simulink model "Sphase"  (R2017a)
settings: Solver=FixedStepDiscrete  StartTime=0.0  StopTime=0.125 - 5e-5  MaxStep=1e-4  RelTol=1e-3
libraries: powerlib x12, auto_lib x2
settings Model: Creator=ioanna  LastModifiedBy=ioanna

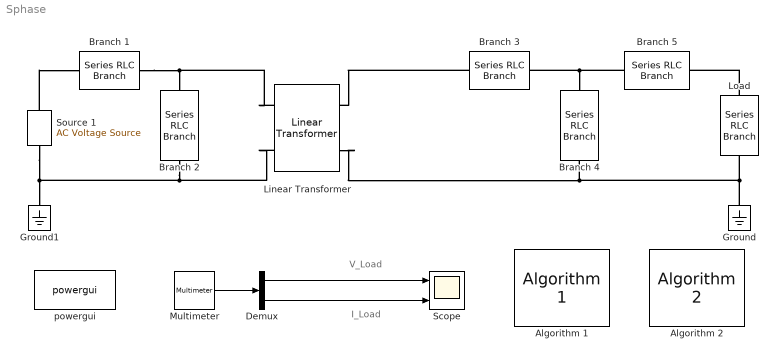
== system Sphase ==
  note: I_Load
  note: V_Load
  Algorithm 1 : auto_lib/Algorithm 1  SystemSampleTime=-1
      settings: SourceProductName=Auto_Design_Framework
  Algorithm 2 : auto_lib/Algorithm 2  SystemSampleTime=-1
      settings: SourceProductName=Auto_Design_Framework
  Branch 1 : powerlib/Elements/Series RLC Branch  LConnTagsString=__new0  RConnTagsString=__new0  BranchType=R  Resistance=5  Inductance=0.02  SetiL0=off  InitialCurrent=0  Capacitance=1e-6  Setx0=off  InitialVoltage=0  Measurements=None
  Branch 2 : powerlib/Elements/Series RLC Branch  LConnTagsString=__new0  RConnTagsString=__new0  BranchType=RC  Resistance=5  Inductance=0.02  SetiL0=off  InitialCurrent=0  Capacitance=1e-4  Setx0=off  InitialVoltage=0  Measurements=None
  Branch 3 : powerlib/Elements/Series RLC Branch  LConnTagsString=__new0  RConnTagsString=__new0  BranchType=R  Resistance=5  Inductance=0.02  SetiL0=off  InitialCurrent=0  Capacitance=1e-6  Setx0=off  InitialVoltage=0  Measurements=None
  Branch 4 : powerlib/Elements/Series RLC Branch  LConnTagsString=__new0  RConnTagsString=__new0  BranchType=RC  Resistance=5  Inductance=0.02  SetiL0=off  InitialCurrent=0  Capacitance=1e-4  Setx0=off  InitialVoltage=0  Measurements=None
  Branch 5 : powerlib/Elements/Series RLC Branch  LConnTagsString=__new0  RConnTagsString=__new0  BranchType=RL  Resistance=5  Inductance=0.02  SetiL0=off  InitialCurrent=0  Capacitance=1e-6  Setx0=off  InitialVoltage=0  Measurements=None
  Demux : Demux  Outputs=2
  Ground : powerlib/Elements/Ground  LConnTagsString=a
  Ground1 : powerlib/Elements/Ground  LConnTagsString=a
  Linear Transformer : powerlib/Elements/Linear Transformer  UNITS=SI  NominalPower=[5e3 50]  winding1=[220 0.5 0.001]  winding2=[440 1 0.002]  ThreeWindings=off  winding3=[3.15e+05 315.06 0.10641]  RmLm=[1e4 50]  Measurements=None  DataType=on
  Load : powerlib/Elements/Series RLC Branch  LConnTagsString=__new0  RConnTagsString=__new0  BranchType=R  Resistance=20  Inductance=0.02  SetiL0=off  InitialCurrent=0  Capacitance=1e-6  Setx0=off  InitialVoltage=0  Measurements=Branch voltage and current
  Multimeter : powerlib/Measurements/Multimeter  PhasorSimulation=off  OutputType=Complex  sel=[1 2]  L=2  Gain=[1 1]  yselected={'Ub: Load','Ib: Load'};  PSBOutputType=1  PSBequivalent=0  AxesSetting=[0,0.1,-100,100]  Display=0  SavedBlockNames=-11
  Scope : Scope  NumInputPorts=2
  Source 1 : powerlib/Electrical Sources/AC Voltage Source  Amplitude=110  Phase=0  Frequency=50  SampleTime=0  Measurements=None  BusType=swing  Pref=10e3  Qref=0  Qmin=-inf  Qmax=+inf
  powergui : powerlib/powergui  Priority=1  SimulationMode=Discrete  SampleTime=50e-6  frequency=60  Iterations=50  frequencyindice=50  Pbase=100e6  ErrMax=1e-4  UnitsV=kV  UnitsW=MW  buscounter=0  FunctionMessages=off  echomessages=off  EnableUseOfTLC=off  CurrentSourceSwitches=off  DisableSnubberDevices=off  DisableRonSwitches=off  DisableVfSwitches=off  DisplayEquations=off  SolverType=Tustin  Interpol=off  ExternalGateDelay=off  methode=off  Ts=100  x0status=zero  SPID=on  SwTol=0  HookPort=off  RestoreLinks=warning  ResistiveCurrentMeasurement=off  Frange=[0:2:500]  Ylog=off  Xlog=on  ShowGrid=off  save=off  variable=ZData  structure=logsout  ZoomFFT=off  StartTime=0.0  cycles=1  DisplayStyle=1  fundamental=60  FreqAxis=off  MaxFrequency=1000  frequencyindicesteady=1  RmsSteady=1  display=off
  wires:
  Multimeter/1 -> Demux/1
  Demux/2 -> Scope/2
  Demux/1 -> Scope/1
  connections:
  Branch 1/LConn1 -- Linear Transformer/LConn1 -- Branch 2/LConn1
  Branch 5/RConn1 -- Branch 3/LConn1 -- Branch 4/LConn1
  Linear Transformer/LConn2 -- Source 1/LConn1 -- Ground1/LConn1 -- Branch 2/RConn1
  Load/LConn1 -- Branch 5/LConn1
  Source 1/RConn1 -- Branch 1/RConn1
  Ground/LConn1 -- Linear Transformer/RConn2 -- Branch 4/RConn1 -- Load/RConn1
  Branch 3/RConn1 -- Linear Transformer/RConn1
